simulink model "fullLoop"  (R2016a)
settings: Solver=FixedStepDiscrete  StartTime=0.0  StopTime=2169  FixedStep=1  RelTol=1e-3
undefined symbols (not defined in the file or in its folder): a, DiscIntNeverNeededParam, mu, sigma
settings Model: Creator=pablo  LastModifiedBy=pai7
settings GRTTargetCC: GeneratePreprocessorConditionals=Use local settings

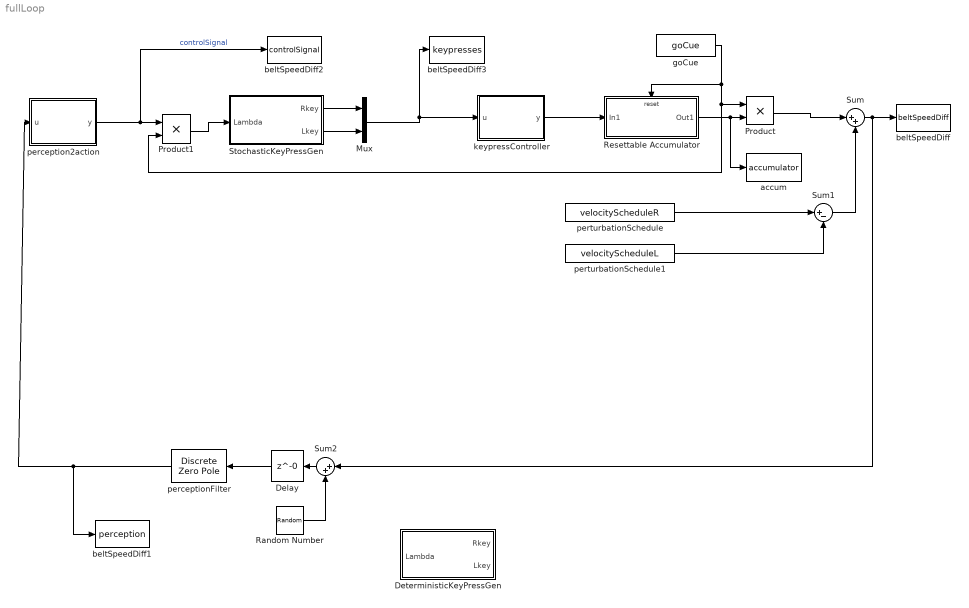
== system fullLoop ==
  Delay : Delay  DelayLength=0
  DeterministicKeyPressGen : Subsystem
  Mux : Mux  Inputs=2
  Product : Product
  Product1 : Product
  Random Number : RandomNumber  Mean=mu  Variance=sigma  Seed=randi(10)  SampleTime=1
  Resettable Accumulator : Subsystem  TreatAsAtomicUnit=on
  StochasticKeyPressGen : Subsystem
  Sum : Sum  Inputs=|++
  Sum1 : Sum  Inputs=|+-
  Sum2 : Sum  Inputs=|++
  accum : ToWorkspace  VariableName=accumulator  SaveFormat=Timeseries  SampleTime=-1
  beltSpeedDiff : ToWorkspace  VariableName=beltSpeedDiff  SaveFormat=Timeseries  SampleTime=-1
  beltSpeedDiff1 : ToWorkspace  VariableName=perception  SaveFormat=Timeseries  SampleTime=-1
  beltSpeedDiff2 : ToWorkspace  VariableName=controlSignal  SaveFormat=Timeseries  SampleTime=-1
  beltSpeedDiff3 : ToWorkspace  VariableName=keypresses  SaveFormat=Timeseries  SampleTime=-1
  goCue : FromWorkspace  VariableName=goCue  OutDataTypeStr=double  SampleTime=0
  keypressController : MATLAB Function  TreatAsAtomicUnit=on
  perception2action : MATLAB Function  TreatAsAtomicUnit=on
  perceptionFilter : DiscreteZeroPole  Zeros=[0]  Poles=[a]  Gain=(1-a)
  perturbationSchedule : FromWorkspace  VariableName=velocityScheduleR  SampleTime=0
  perturbationSchedule1 : FromWorkspace  VariableName=velocityScheduleL  SampleTime=0
  wires:
  Sum/1 -> Sum2/1, beltSpeedDiff/1
  perceptionFilter/1 -> perception2action/1(u), beltSpeedDiff1/1
  goCue/1 -> Product1/2, Product/1, Resettable Accumulator/Reset
  Delay/1 -> perceptionFilter/1
  Random Number/1 -> Sum2/2
  keypressController/1(y) -> Resettable Accumulator/1(In1)
  Mux/1 -> keypressController/1(u), beltSpeedDiff3/1
  Product/1 -> Sum/1
  Resettable Accumulator/1(Out1) -> accum/1, Product/2
  Sum2/1 -> Delay/1
  StochasticKeyPressGen/1(Rkey) -> Mux/1
  StochasticKeyPressGen/2(Lkey) -> Mux/2
  perturbationSchedule/1 -> Sum1/1
  perturbationSchedule1/1 -> Sum1/2
  Sum1/1 -> Sum/2
  Product1/1 -> StochasticKeyPressGen/1(Lambda)
  perception2action/1(y) -> Product1/1, beltSpeedDiff2/1  "controlSignal"

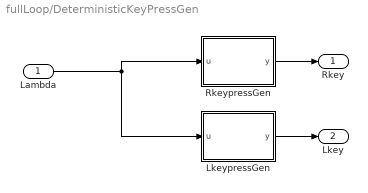
== system fullLoop/DeterministicKeyPressGen ==
  Lambda : Inport
  LkeypressGen : MATLAB Function  TreatAsAtomicUnit=on
  RkeypressGen : MATLAB Function  TreatAsAtomicUnit=on
  Rkey : Outport
  Lkey : Outport  Port=2
  wires:
  Lambda/1 -> LkeypressGen/1(u), RkeypressGen/1(u)
  RkeypressGen/1(y) -> Rkey/1
  LkeypressGen/1(y) -> Lkey/1

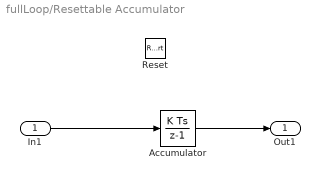
== system fullLoop/Resettable Accumulator ==
  In1 : Inport
  Reset : ResetPort  DisableCoverage=on  ResetTriggerType=either  PropagateVarSize=During execution
  Accumulator : DiscreteIntegrator  ICPrevOutput=DiscIntNeverNeededParam  ICPrevScaledInput=DiscIntNeverNeededParam
  Out1 : Outport
  wires:
  In1/1 -> Accumulator/1
  Accumulator/1 -> Out1/1

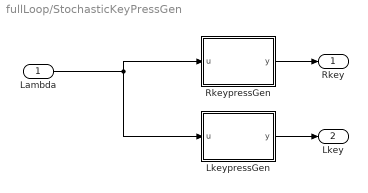
== system fullLoop/StochasticKeyPressGen ==
  Lambda : Inport
  LkeypressGen : MATLAB Function  TreatAsAtomicUnit=on
  RkeypressGen : MATLAB Function  TreatAsAtomicUnit=on
  Rkey : Outport
  Lkey : Outport  Port=2
  wires:
  Lambda/1 -> LkeypressGen/1(u), RkeypressGen/1(u)
  RkeypressGen/1(y) -> Rkey/1
  LkeypressGen/1(y) -> Lkey/1

== matlab function fullLoop/StochasticKeyPressGen/LkeypressGen ==
  data: u input; y output
function y = fcn(u)
%#codegen

if sign(u)==-1
    y = poissrnd(-u);
else
    y=0;
end

== matlab function fullLoop/StochasticKeyPressGen/RkeypressGen ==
  data: u input; y output
function y = fcn(u)
%#codegen

if sign(u)==1
    y = poissrnd(u);
else
    y=0;
end

== matlab function fullLoop/keypressController ==
  data: u input; y output size=1
function y = fcn(u)
%#codegen

actionRange=[6 10];

u(u>7)=7;
R=randi(actionRange,7,1); %Not allowing more than 7 keypresses. 
%This way to limit rate is very inefficient but required by simulink for static mem allocation
L=randi(actionRange,7,1);

y=sum(R(1:u(1)))-sum(L(1:u(2)));
end

== matlab function fullLoop/perception2action ==
  data: u input; y output size=1
function y = fcn(u)
%#codegen
map=1;
k=-5/200;
th=50;
A=5/exp(5);
switch map
    case 1
%Linear map:
y=k*u;

    case 2
%Linear with threshold:
y= k*(abs(u)-th)*(abs(u)>th)*sign(u);

    case 3
%Quadratic map:
y=(k/200)*u^2;

    case 4
y=A*exp(k*u);

end

end

== matlab function fullLoop/DeterministicKeyPressGen/LkeypressGen ==
  data: u input; y output
function y = fcn(u)
%#codegen

if sign(u)==-1
    y = round(-u);
else
    y=0;
end

== matlab function fullLoop/DeterministicKeyPressGen/RkeypressGen ==
  data: u input; y output
function y = fcn(u)
%#codegen

if sign(u)==1
    y = round(u);
else
    y=0;
end
